simulink model "state_space"  (R2019a)
settings: Solver=VariableStepAuto  StartTime=0.0  StopTime=10.0  RelTol=1e-3
settings Model: Creator=harkib  LastModifiedBy=harki
settings DataIOCC: ReturnWorkspaceOutputs=off
settings DebuggingCC: ArithmeticOperatorsInVariantConditions=warning
settings SFSimCC: SimUseLocalCustomCode=off
settings RTWCC: RTWUseLocalCustomCode=off

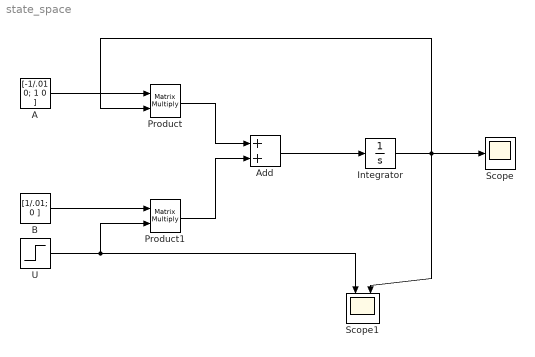
== system state_space ==
  A : Constant  Value=[-1/.01 0; 1 0 ]
  Add : Sum
  B : Constant  Value=[1/.01; 0 ]
  Integrator : Integrator
  Product : Product  Multiplication=Matrix(*)
  Product1 : Product  Multiplication=Matrix(*)
  Scope : Scope
  Scope1 : Scope  NumInputPorts=2
  U : Step  SampleTime=0
  wires:
  Add/1 -> Integrator/1
  Product1/1 -> Add/2
  Product/1 -> Add/1
  B/1 -> Product1/1
  U/1 -> Scope1/1, Product1/2
  A/1 -> Product/1
  Integrator/1 -> Scope1/2, Scope/1, Product/2
